simulink model "Tuning_retta"  (R2015a)
settings: Solver=ode3  StartTime=0.0  StopTime=inf  FixedStep=1e-3  RelTol=1e-3
values from neighbouring files (symbols this model uses):
  conversion_V2mm = 17.8/(3540-260)    (= 0.00542682926829)    [Datasheet.m]    (also in setup.m)
undefined symbols (not defined in the file or in its folder): fdesignblkfcn, gcbh
libraries: PoliArd x6, dspswit3 x1, simulink x1
settings Model: ExtModeTrigDuration=2  Creator=User  LastModifiedBy=User
settings SolverCC: AutoInsertRateTranBlk=on
settings OptimizationCC: OptimizeModelRefInitCode=on  LifeSpan=1
settings DebuggingCC: UnderspecifiedInitializationDetection=Classic  MergeDetectMultiDrivingBlocksExec=none
settings HardwareCC: ProdLargestAtomicInteger=Long  ProdLargestAtomicFloat=Double  ProdEndianess=LittleEndian  ProdHWDeviceType=ARM Compatible->ARM Cortex
settings RTWCC: SystemTargetFile=realtime.tlc  GenerateMakefile=off  TemplateMakefile=realtime.tmf  Description=Run on Target Hardware  RTWVerbose=off
settings ERTTargetCC: CombineOutputUpdateFcns=off  ExtModeTransport=3  ExtModeMexFile=ext_serial_win32_comm_rtt  ExtModeMexArgs=0 1 9600  ERTSrcFileBannerTemplate=realtime_code_template.cgt  ERTHdrFileBannerTemplate=realtime_code_template.cgt  ERTDataSrcFileTemplate=realtime_code_template.cgt  ERTDataHdrFileTemplate=realtime_code_template.cgt  ERTCustomFileTemplate=realtime_file_process.tlc

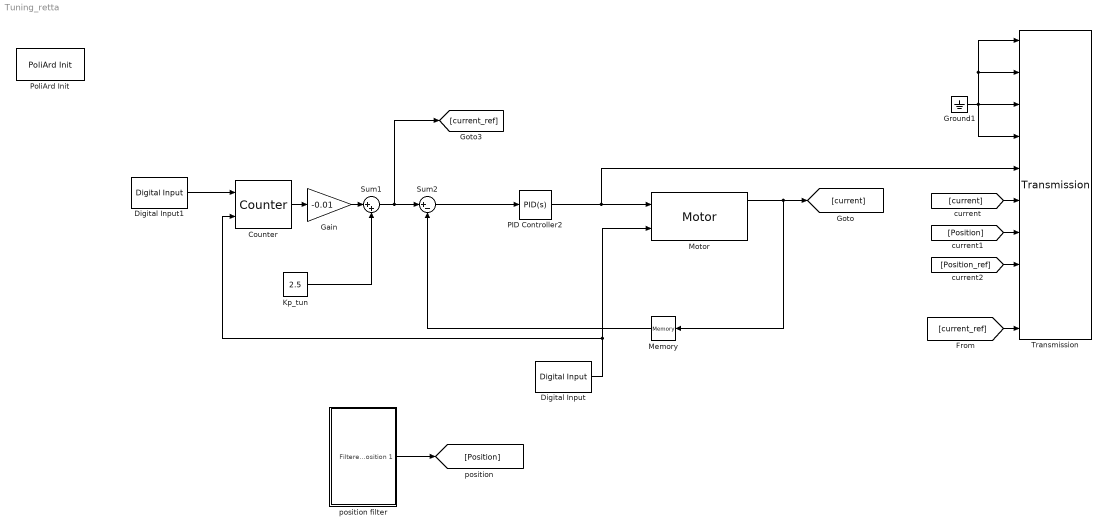
== system Tuning_retta ==
  Counter : dspswit3/Counter  Direction=Up  CountEvent=Either edge  CounterSize=User defined  MaxCount=10000  InitialCount=0  Output=Count  HitValue=32  ResetInput=on  SamplesPerFrame=1  Ts=1  CntDtype=double  HitDtype=Logical
  Digital Input : PoliArd/Digital Input  DI_pin=3  DIsample=-1
  Digital Input1 : PoliArd/Digital Input  DI_pin=2  DIsample=-1
  Gain : Gain  Gain=-0.01
  Ground1 : Ground
  "Kp_tun " : Constant  Value=2.5
  Memory : Memory
  Motor : PoliArd/Motor  MotorID=2  DC_bus_mask=24  dt_mot=-1
  PID Controller2 : simulink/Continuous/PID Controller  Controller=PID  TimeDomain=Continuous-time  SampleTime=-1  IntegratorMethod=Forward Euler  FilterMethod=Forward Euler  Form=Parallel  UseFilter=on  ControllerParametersSource=internal  P=24.75  I=697  D=0  N=0  InitialConditionSource=internal  InitialConditionForIntegrator=0  InitialConditionForFilter=0  ExternalReset=none  LimitOutput=on  UpperSaturationLimit=24  LowerSaturationLimit=-24  LinearizeAsGain=on  AntiWindupMode=none  Kb=1  TrackingMode=off  Kt=1  PParamMin=[]  PParamMax=[]  IParamMin=[]  IParamMax=[]  DParamMin=[]  DParamMax=[]  NParamMin=[]  NParamMax=[]  KbParamMin=[]  KbParamMax=[]  KtParamMin=[]  KtParamMax=[]  POutMin=[]  POutMax=[]  IOutMin=[]  IOutMax=[]  DOutMin=[]  DOutMax=[]  NOutMin=[]  NOutMax=[]  KbOutMin=[]  KbOutMax=[]  KtOutMin=[]  KtOutMax=[]  IntegratorOutMin=[]  IntegratorOutMax=[]  FilterOutMin=[]  FilterOutMax=[]  SumOutMin=[]  SumOutMax=[]  SumI1OutMin=[]  SumI1OutMax=[]  SumI2OutMin=[]  SumI2OutMax=[]  SumI3OutMin=[]  SumI3OutMax=[]  SumDOutMin=[]  SumDOutMax=[]  SaturationOutMin=[]  SaturationOutMax=[]  IntegratorContinuousStateAttributes=''  IntegratorStateMustResolveToSignalObject=off  IntegratorRTWStateStorageClass=Auto  FilterContinuousStateAttributes=''  FilterStateMustResolveToSignalObject=off  FilterRTWStateStorageClass=Auto  DifferentiatorICPrevScaledInput=0  DifferentiatorOutMin=[]  DifferentiatorOutMax=[]
  PoliArd Init : PoliArd/PoliArd Init
  Sum1 : Sum  Inputs=|++
  Sum2 : Sum  Inputs=|+-
  Transmission : PoliArd/Transmission  sample_freq=100  sig_to_send=6
  position filter : Subsystem
  wires:
  Motor/1 -> [current], Memory/1
  position filter/1(Filtered position 1) -> [Position]
  Sum2/1 -> PID Controller2/1
  Ground1/1 -> Transmission/3, Transmission/1, Transmission/2, Transmission/4
  Digital Input/1 -> Motor/2, Counter/2
  Memory/1 -> Sum2/2
  PID Controller2/1 -> Transmission/5, Motor/1
  [current] -> Transmission/6
  [Position] -> Transmission/7
  [Position_ref] -> Transmission/8
  [current_ref] -> Transmission/10
  Digital Input1/1 -> Counter/1
  Counter/1 -> Gain/1
  "Kp_tun "/1 -> Sum1/2
  Gain/1 -> Sum1/1
  Sum1/1 -> [current_ref], Sum2/1

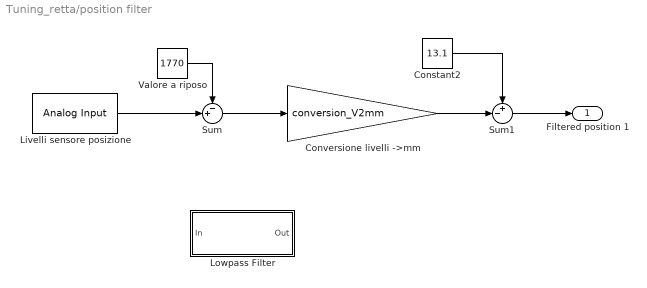
== system Tuning_retta/position filter ==
  Constant2 : Constant  Value=13.1
  Conversione livelli ->mm : Gain  Gain=conversion_V2mm
  "Livelli sensore posizione " : PoliArd/Analog Input  AIpin_mask=2  AIsample=-1
  Lowpass Filter : Subsystem  DialogController=fdesignblkfcn  InitFcn=fdesignblkfcn(gcbh, {'InitFcn'});  mask(Lowpass Filter){}
      mask help: Design a lowpass filter
      settings: CopyFcn=fdesignblkfcn(gcbh, {'CopyFcn'});
      mask Help: helpview(mapfilelocation('dsp'), 'dsplowpassfilter');
      mask Display: disp('Lowpass')
  Sum : Sum  Inputs=-+|
  Sum1 : Sum  Inputs=+-|
  Valore a riposo : Constant  Value=1770
  Filtered position 1 : Outport
  wires:
  Sum1/1 -> Filtered position 1/1
  Constant2/1 -> Sum1/1
  Conversione livelli ->mm/1 -> Sum1/2
  Valore a riposo/1 -> Sum/1
  Sum/1 -> Conversione livelli ->mm/1
  "Livelli sensore posizione "/1 -> Sum/2

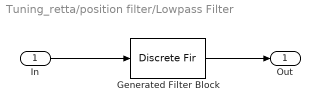
== system Tuning_retta/position filter/Lowpass Filter ==
  In : Inport
  Generated Filter Block : DiscreteFir  Tag=BlockMethodSubSystem  Coefficients=[-0.096626420854236783 0.24327035766280955 0.68025369464798469 0.24327035766280955 -0.096626420854236783]  InputProcessing=Columns as channels (frame based)
  Out : Outport
  wires:
  Generated Filter Block/1 -> Out/1
  In/1 -> Generated Filter Block/1
